simulink model "buckconverter"  (R2023b)
settings: Solver=ode23t  StartTime=0.0  StopTime=15  RelTol=1e-3
undefined symbols (not defined in the file): Ion, Lithium
libraries: spsSeriesRLCBranchLib x3, spsBatteryLib x1, spsDiodeLib x1, spsMosfetLib x1, spsPVArrayLib x1, simulink x1, sps_lib x1
settings Model: Creator=ASUS  LastModifiedBy=ASUS
settings DebuggingCC: SignalInfNanChecking=error

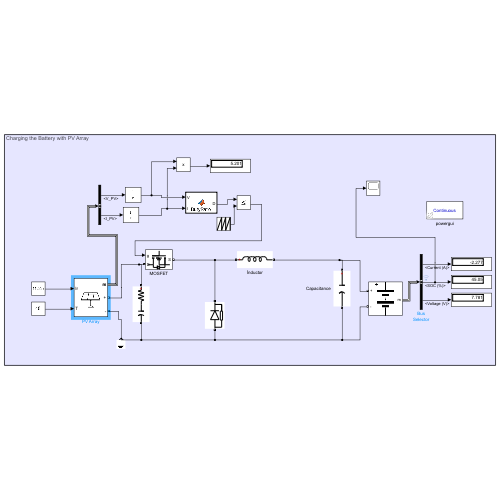
[thumbnail: Simulink's stored preview of the top-level diagram]
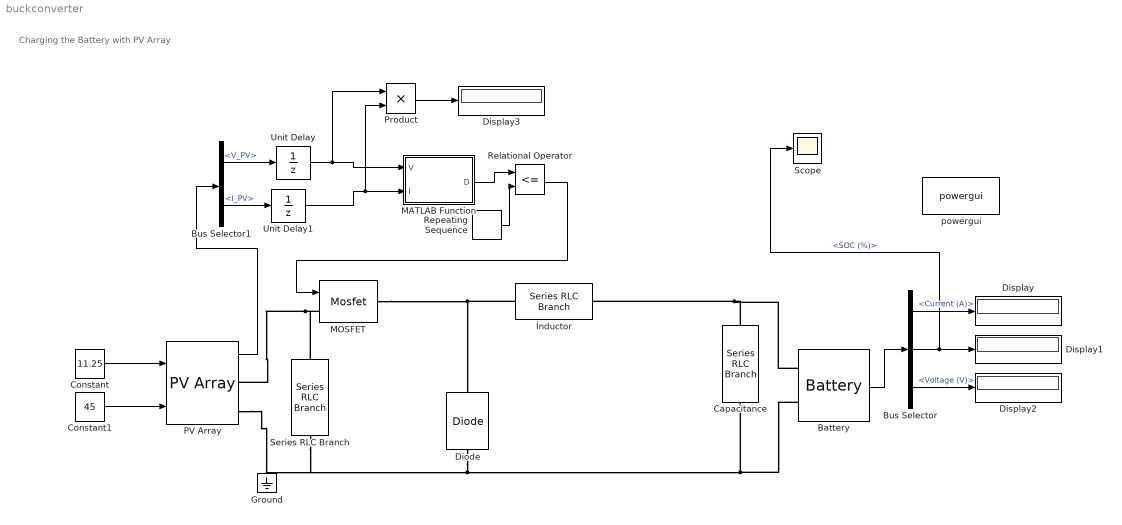
== system buckconverter ==
  note: Charging the Battery with PV Array
  Battery : spsBatteryLib/Battery  BatType=Lithium-Ion  ShowTempParam=off  ThermalPreset=no  ShowAgeParam=off  NomV=7.2  NomQ=6  SOC=45  Batt_Tr=1  PresetModel=on  MaxQ=6  MinV=5.4  FullV=8.3807  Dis_rate=2.6087  R=0.012  Normal_OP=5.4261  expZone="[7.7788     0.29478]"  current=[6.5 13 32.5]  Units=Time  Tci=20  NomT=20  T2=-30  MaxQ2=4.8  FullV2=7.1  Normal_OP2=5.655  expZone2="[6.58           1]"  Rca=0.6  ti=2000  Dp=0  Neq0=0  Tsim=1e6  Ta1=25  Qeol=5.4*0.9  Reol=0.013333*1.2  Char_age=[2.3478, 3]  Dis_age=[2.3478, 10]  N1=1500  N2=10500  N3=1000  N4=1400  Ta2=45  N5=950
  Bus Selector : BusSelector  OutputSignals=Current (A),SOC (%),Voltage (V)
  Bus Selector1 : BusSelector  OutputSignals=V_PV,I_PV
  Capacitance : spsSeriesRLCBranchLib/Series RLC Branch  LConnTagsString=__new0  RConnTagsString=__new0  BranchType=C  Resistance=1  Inductance=1e-3  SetiL0=off  InitialCurrent=0  Capacitance=85e-6  Setx0=off  InitialVoltage=0  Measurements=None
  Constant : Constant  Value=11.25  SampleTime=10
  Constant1 : Constant  Value=45
  Diode : spsDiodeLib/Diode  Ron=0.001  Lon=0  Vf=0.3  IC=0  UseSnubber=0  Rs=500  Cs=250e-9  Measurements=off
  Display{,1..3} (4 alike) : Display
  Ground : Ground
  MATLAB Function : MATLAB Function  TreatAsAtomicUnit=on
  MOSFET : spsMosfetLib/Mosfet  Ron=0.005  Lon=0  Rd=0.01  Vfd=0  IC=0  Rs=1e5  Cs=inf  Measurements=off
  PV Array : spsPVArrayLib/PV Array  Npar=6  Nser=10  PlotType=array @ 1000 W/m2 & specified temperatures  S_vec="[ 1000  500  100 ]"  Temp_C_vec="[ 45 25  ]"  ModuleName=AXITEC AC-250M/156-60S  PlotWhenSelected=off  Pm=249.888  Ncell=60  Voc=37.51  Isc=8.88  Vm=30.4  Im=8.22  beta_Voc_pc=-0.323  alpha_Isc_pc=0.065  beta_Voc=-0.12116  alpha_Isc=0.005772  IL=8.982  I0=7.7479e-11  nI=0.95689  Rsh=90.6925  Rs=0.32417  RobustModel=off  RobustCellTemperature=313.3991  BAL=on  Tc=1e-6  Tfilter=5e-5
  Product : Product
  Relational Operator : RelationalOperator  Operator=<=  OutDataTypeStr=boolean  RndMeth=Simplest  InputSameDT=off
  Repeating Sequence : simulink/Sources/Repeating Sequence  rep_seq_t=[0 0.0002]  rep_seq_y=[0 1]
  Scope : Scope
  Series RLC Branch : spsSeriesRLCBranchLib/Series RLC Branch  LConnTagsString=__new0  RConnTagsString=__new0  BranchType=RC  Resistance=0.0001  Inductance=1e-3  SetiL0=off  InitialCurrent=0  Capacitance=1000e-6  Setx0=off  InitialVoltage=0  Measurements=None
  Unit Delay : UnitDelay  SampleTime=1e-4  HasFrameUpgradeWarning=on
  Unit Delay1 : UnitDelay  SampleTime=1e-4  HasFrameUpgradeWarning=on
  powergui : sps_lib/powergui  Priority=1  SimulationMode=Continuous  SampleTime=1e-6  frequency=60  Iterations=50  frequencyindice=0  Pbase=100e6  ErrMax=1e-4  UnitsV=kV  UnitsW=MW  buscounter=0  FunctionMessages=off  echomessages=off  EnableUseOfTLC=off  CurrentSourceSwitches=off  DisableSnubberDevices=off  DisableRonSwitches=off  DisableVfSwitches=off  DisplayEquations=off  AutomaticDiscreteSolvers=off  SolverType=Tustin/Backward Euler (TBE)  Interpol=off  ExternalGateDelay=off  methode=off  Ts=100  x0status=blocks  SPID=on  SwTol=0  HookPort=off  NonlinearTolerance=1e-4  nMaxIteration=100  ContinueOnMaxIteration=off  RestoreLinks=warning  ResistiveCurrentMeasurement=off  Frange=[0:2:500]  Ylog=off  Xlog=on  ShowGrid=off  save=off  variable=ZData  structure=0  ZoomFFT=off  StartTime=0.0  cycles=1  DisplayStyle=1  fundamental=60  FreqAxis=off  MaxFrequency=1000  frequencyindicesteady=1  RmsSteady=1  display=off
  İnductor : spsSeriesRLCBranchLib/Series RLC Branch  LConnTagsString=__new0  RConnTagsString=__new0  BranchType=L  Resistance=0  Inductance=34.5e-6  SetiL0=off  InitialCurrent=0  Capacitance=0  Setx0=off  InitialVoltage=0  Measurements=None
  wires:
  Constant/1 -> PV Array/1
  Constant1/1 -> PV Array/2
  Battery/1 -> Bus Selector/1
  Bus Selector/1 -> Display/1  "<Current (A)>"
  Bus Selector/2 -> Scope/1, Display1/1  "<SOC (%)>"
  Bus Selector/3 -> Display2/1  "<Voltage (V)>"
  PV Array/1 -> Bus Selector1/1
  Bus Selector1/1 -> Unit Delay/1  "<V_PV>"
  Bus Selector1/2 -> Unit Delay1/1  "<I_PV>"
  Unit Delay/1 -> Product/1, MATLAB Function/1(V)
  Unit Delay1/1 -> Product/2, MATLAB Function/2(I)
  MATLAB Function/1(D) -> Relational Operator/1
  Repeating Sequence/1 -> Relational Operator/2
  Relational Operator/1 -> MOSFET/1
  Product/1 -> Display3/1
  connections:
  İnductor/LConn1 -- MOSFET/RConn1 -- Diode/RConn1
  Capacitance/LConn1 -- Battery/LConn1 -- İnductor/RConn1
  Diode/LConn1 -- Series RLC Branch/RConn1 -- PV Array/RConn2 -- Capacitance/RConn1 -- Battery/LConn2
  MOSFET/LConn1 -- Series RLC Branch/LConn1 -- PV Array/RConn1

== matlab function buckconverter/MATLAB Function ==
  data: V input; D output; I input
function D = DutyRatio(V,I)

Dmax=0.47;
Dmin=0;
Dinit=0.47;
deltaD=0.001;
persistent Vold Pold Dold;

dataType= 'double';

if isempty(Vold)
    Vold=0;
    Pold=0;
    Dold=Dinit;
end

P=V*I;
dV=V-Vold;
dP=P-Pold;

if dP  ~=0
    if dP<0
        if dV<0
           D=Dold+deltaD;
        else
            D=Dold-deltaD;
        end
    else
        if dV<0
           D=Dold+deltaD;
        else 
            D=Dold-deltaD;
        end 
    end 
else D=Dold;
end
if D>= Dmax| D<=Dmin
    D=Dold;
end
Dold=D;
Vold=V;
Pold=P;
